simulink model "Lab2"  (R2023b)
settings: Solver=VariableStepAuto  StartTime=0.0  StopTime=10  RelTol=1e-3
settings Model: Creator=gaafa  LastModifiedBy=gaafa

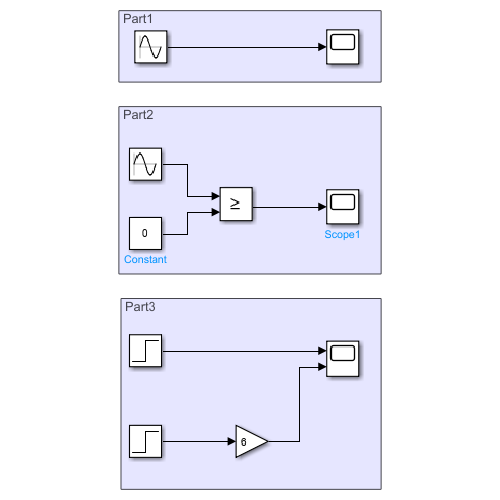
[thumbnail: Simulink's stored preview of the top-level diagram]
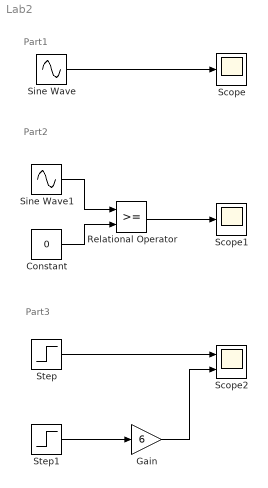
== system Lab2 ==
  note: Part3
  note: Part1
  note: Part2
  Constant : Constant  Value=0
  Gain : Gain  Gain=6
  Relational Operator : RelationalOperator  OutDataTypeStr=boolean  RndMeth=Simplest  InputSameDT=off
  Scope : Scope
  Scope1 : Scope
  Scope2 : Scope  NumInputPorts=2
  Sine Wave : Sin  Frequency=2*pi*1  SampleTime=0
  Sine Wave1 : Sin  Frequency=2*pi*1  SampleTime=0
  Step : Step  Time=0  SampleTime=0
  Step1 : Step  Time=2  SampleTime=0
  wires:
  Sine Wave/1 -> Scope/1
  Sine Wave1/1 -> Relational Operator/1
  Constant/1 -> Relational Operator/2
  Relational Operator/1 -> Scope1/1
  Step/1 -> Scope2/1
  Step1/1 -> Gain/1
  Gain/1 -> Scope2/2
